simulink model "sl_subsys_for1"  (Simulink 6.0)
settings: Solver=FixedStepDiscrete  StartTime=0.0  StopTime=10.0  FixedStep=1  RelTol=1e-3
settings Model: CovMetricSettings=d  Creator=The MathWorks Inc.  LastModifiedBy=batserve  ExtModeAutoUpdateStatusClock=off
settings OptimizationCC: BlockReduction=off  BooleanDataType=off
settings DebuggingCC: CheckExecutionContextPreStartOutputMsg=on  CheckExecutionContextRuntimeOutputMsg=on  SolverPrmCheckMsg=none
settings HardwareCC: TargetUnknown=on

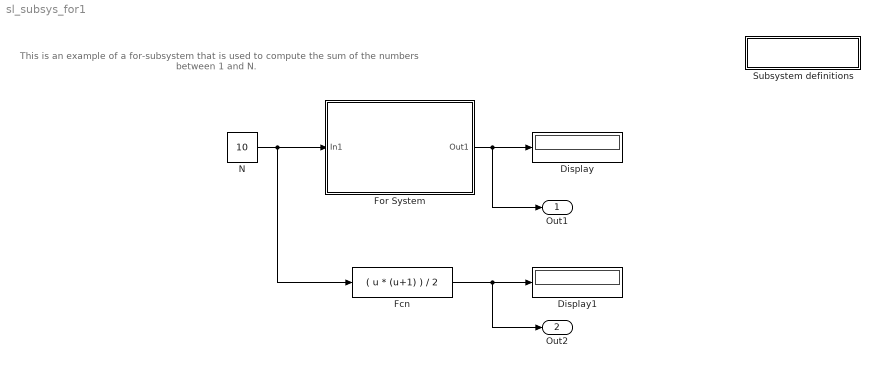
== system sl_subsys_for1 ==
  note: This is an example of a for-subsystem that is used
      | to compute the sum of the numbers between 1 and N.
  " Subsystem definitions" : Subsystem  PropExecContextAcrossSSBoundary=on
      settings: OpenFcn=helpview([matlabroot,'/toolbox/simulink/simdemos/sl_subsys_definitions.html']);
      mask Display: disp('Subsystem\ndefinitions')
  Display : Display
  Display1 : Display
  Fcn : Fcn  Expr=( u * (u+1) ) / 2
  For System : Subsystem  TreatAsAtomicUnit=on  PropExecContextAcrossSSBoundary=on
  N : Constant  Value=10
  Out1 : Outport
  Out2 : Outport  Port=2
  wires:
  N/1 -> For System/1(In1), Fcn/1
  For System/1(Out1) -> Display/1, Out1/1
  Fcn/1 -> Display1/1, Out2/1

== system sl_subsys_for1/ Subsystem definitions ==

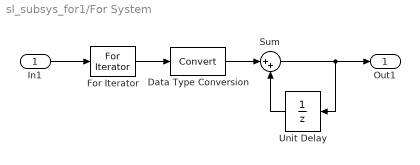
== system sl_subsys_for1/For System ==
  In1 : Inport  Port=1  LatchInput=off
  Data Type Conversion : DataTypeConversion  OutDataTypeMode=double  SaturateOnIntegerOverflow=on  RndMeth=Zero
  For Iterator : ForIterator  ResetStates=reset  IterationSource=external
  Sum : Sum  Inputs=|++  SaturateOnIntegerOverflow=on  InputSameDT=on
  Unit Delay : UnitDelay  Orientation=left  SampleTime=-1
  Out1 : Outport
  wires:
  Sum/1 -> Unit Delay/1, Out1/1
  For Iterator/1 -> Data Type Conversion/1
  In1/1 -> For Iterator/1
  Unit Delay/1 -> Sum/2
  Data Type Conversion/1 -> Sum/1
